simulink model "position_stabilization"  (R2018b)
settings: Solver=VariableStepAuto  StartTime=0.0  StopTime=10.0  RelTol=1e-3
values from neighbouring files (symbols this model uses):
  g = 9.8    [para.m]
  Ixx = 0.1    [para.m]
  m = 2    [para.m]
  x0 = zeros(6, 1)    [para.m]
settings Model: Creator=arthus  LastModifiedBy=longh

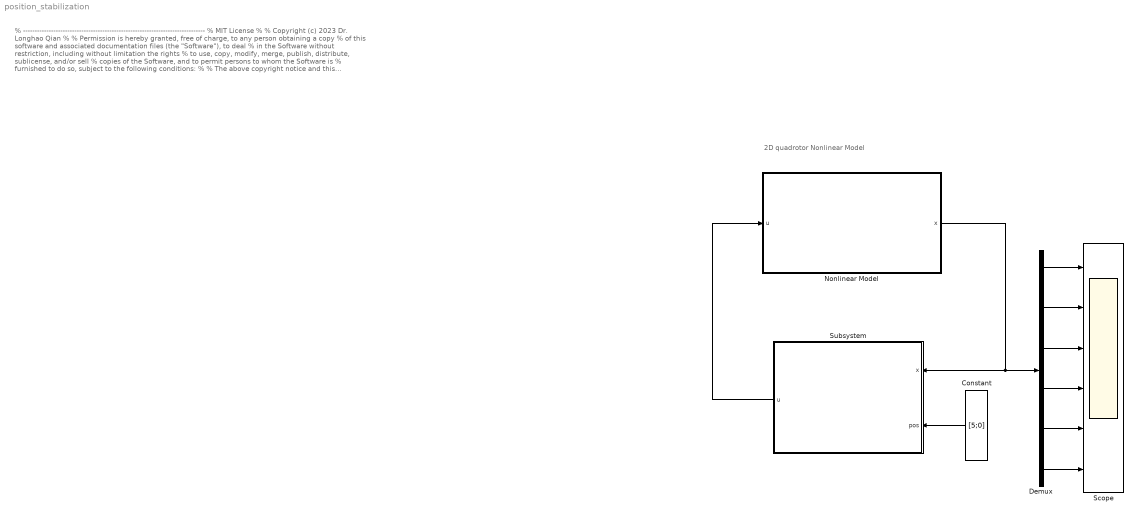
== system position_stabilization ==
  note: % ------------------------------------------------------------------------------
      | % MIT License
      | %
      | % Copyright (c) 2023 Dr. Longhao Qian
      | %
      | % Permission is hereby granted, free of charge, to any person obtaining a copy
      | % of this software and associated documentation files (the "Software"), to deal
      | % in the Software without restriction, including without limitation the rights
      | % to use, copy, modify, merge, publish, distribute, sublicense, and/or sell
      | % copies of the Software, and to permit persons to whom the Software is
      | % furnished to do so, subject to the following conditions:
      | %
      | % The above copyright notice and this permission notice shall be included in all
      | % copies or substantial portions of the Software.
      | %
      | % THE SOFTWARE IS PROVIDED "AS IS", WITHOUT WARRANTY OF ANY KIND, EXPRESS OR
      | % IMPLIED, INCLUDING BUT NOT LIMITED TO THE WARRANTIES OF MERCHANTABILITY,
      | % FITNESS FOR A PARTICULAR PURPOSE AND NONINFRINGEMENT. IN NO EVENT SHALL THE
      | % AUTHORS OR COPYRIGHT HOLDERS BE LIABLE FOR ANY CLAIM, DAMAGES OR OTHER
      | % LIABILITY, WHETHER IN AN ACTION OF CONTRACT, TORT OR OTHERWISE, ARISING FROM,
      | % OUT OF OR IN CONNECTION WITH THE SOFTWARE OR THE USE OR OTHER DEALINGS IN THE
      | % SOFTWARE.
      | % ------------------------------------------------------------------------------
  note: 2D quadrotor Nonlinear Model
  Constant : Constant  Value=[5;0]  VectorParams1D=off
  Demux : Demux  Outputs=6
  Nonlinear Model : Subsystem
  Scope : Scope  NumInputPorts=6
  Subsystem : Subsystem
  wires:
  Nonlinear Model/1(x) -> Subsystem/1(x), Demux/1
  Subsystem/1(u) -> Nonlinear Model/1(u)
  Demux/1 -> Scope/1
  Demux/2 -> Scope/2
  Demux/3 -> Scope/3
  Demux/4 -> Scope/4
  Demux/5 -> Scope/5
  Demux/6 -> Scope/6
  Constant/1 -> Subsystem/2(pos)

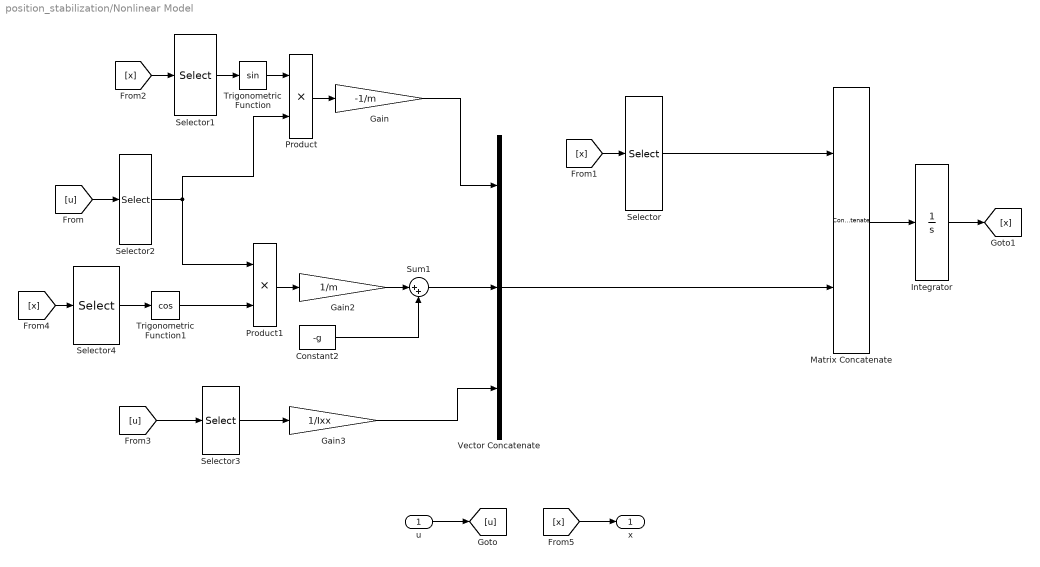
== system position_stabilization/Nonlinear Model ==
  u : Inport
  Constant2 : Constant  Value=-g
  Gain : Gain  Gain=-1/m
  Gain2 : Gain  Gain=1/m
  Gain3 : Gain  Gain=1/Ixx
  Integrator : Integrator  InitialCondition=x0
  Matrix Concatenate : Concatenate  Mode=Multidimensional array
  Product : Product
  Product1 : Product
  Selector : Selector  InputPortWidth=6  IndexOptions=Index vector (dialog)  Indices=[4 5 6]  OutputSizes=1
  Selector1 : Selector  InputPortWidth=6  IndexOptions=Index vector (dialog)  Indices=[3]  OutputSizes=1
  Selector2 : Selector  InputPortWidth=2  IndexOptions=Index vector (dialog)  Indices=[1]  OutputSizes=1
  Selector3 : Selector  InputPortWidth=2  IndexOptions=Index vector (dialog)  Indices=[2]  OutputSizes=1
  Selector4 : Selector  InputPortWidth=6  IndexOptions=Index vector (dialog)  Indices=[3]  OutputSizes=1
  Sum1 : Sum  Inputs=|++
  Trigonometric Function : Trigonometry
  Trigonometric Function1 : Trigonometry  Operator=cos
  Vector Concatenate : Concatenate  NumInputs=3  Mode=Multidimensional array
  x : Outport
  wires:
  Vector Concatenate/1 -> Matrix Concatenate/2
  Gain/1 -> Vector Concatenate/1
  Trigonometric Function/1 -> Product/1
  [x] -> x/1
  Integrator/1 -> [x]
  Product/1 -> Gain/1
  Selector2/1 -> Product1/1, Product/2
  [x] -> Selector4/1
  [u] -> Selector3/1
  [x] -> Selector/1
  Selector4/1 -> Trigonometric Function1/1
  Selector3/1 -> Gain3/1
  Sum1/1 -> Vector Concatenate/2
  Gain3/1 -> Vector Concatenate/3
  Product1/1 -> Gain2/1
  Selector1/1 -> Trigonometric Function/1
  Constant2/1 -> Sum1/2
  Trigonometric Function1/1 -> Product1/2
  [u] -> Selector2/1
  [x] -> Selector1/1
  Selector/1 -> Matrix Concatenate/1
  Matrix Concatenate/1 -> Integrator/1
  Gain2/1 -> Sum1/1
  u/1 -> [u]

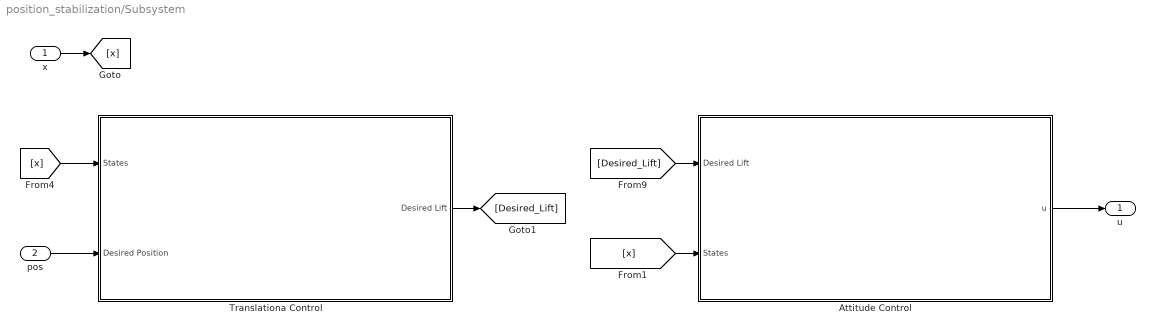
== system position_stabilization/Subsystem ==
  x : Inport
  pos : Inport  Port=2
  Attitude Control : Subsystem
  Translationa Control : Subsystem
  u : Outport
  wires:
  x/1 -> [x]
  [x] -> Attitude Control/2(States)
  pos/1 -> Translationa Control/2(Desired Position)
  [x] -> Translationa Control/1(States)
  Translationa Control/1(Desired Lift) -> [Desired_Lift]
  [Desired_Lift] -> Attitude Control/1(Desired Lift)
  Attitude Control/1(u) -> u/1

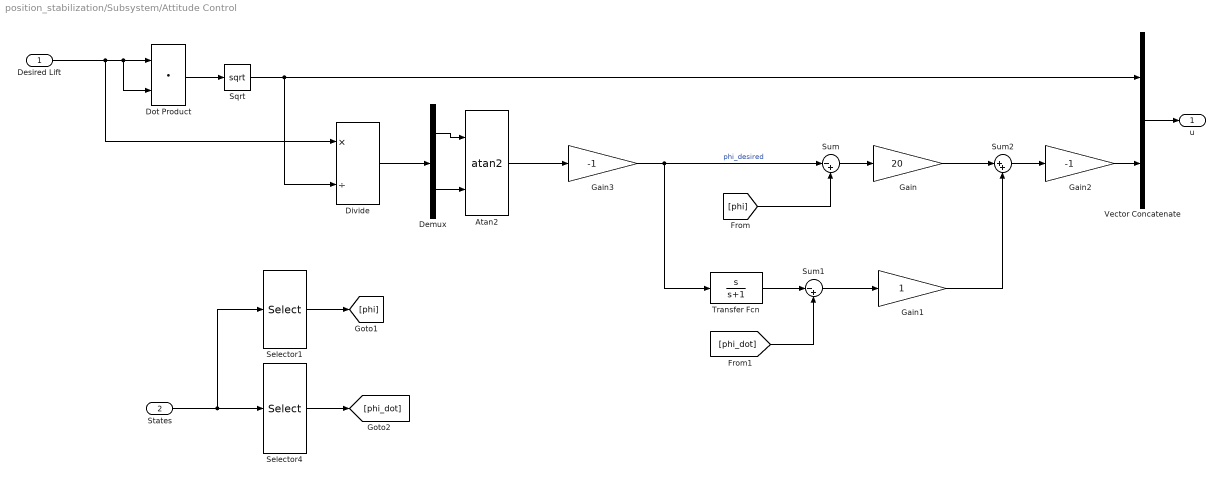
== system position_stabilization/Subsystem/Attitude Control ==
  Desired Lift : Inport
  States : Inport  Port=2
  Atan2 : Trigonometry  Operator=atan2
  Demux : Demux  Outputs=2
  Divide : Product  Inputs=*/
  Dot Product : DotProduct  InputSameDT=on  OutDataTypeStr=Inherit: Inherit via internal rule
  Gain : Gain  Gain=20
  Gain1 : Gain
  Gain2 : Gain  Gain=-1
  Gain3 : Gain  Gain=-1
  Selector1 : Selector  InputPortWidth=6  IndexOptions=Index vector (dialog)  Indices=[3]  OutputSizes=1
  Selector4 : Selector  InputPortWidth=6  IndexOptions=Index vector (dialog)  Indices=[6]  OutputSizes=1
  Sqrt : Sqrt  SaturateOnIntegerOverflow=on
  Sum : Sum  Inputs=|-+
  Sum1 : Sum  Inputs=|-+
  Sum2 : Sum  Inputs=|++
  Transfer Fcn : TransferFcn  Numerator=[1 0]  Denominator=[1 1]
  Vector Concatenate : Concatenate
  u : Outport
  wires:
  Selector1/1 -> [phi]
  States/1 -> Selector4/1, Selector1/1
  Selector4/1 -> [phi_dot]
  Desired Lift/1 -> Divide/1, Dot Product/2, Dot Product/1
  Dot Product/1 -> Sqrt/1
  Sqrt/1 -> Divide/2, Vector Concatenate/1
  Vector Concatenate/1 -> u/1
  Divide/1 -> Demux/1
  Atan2/1 -> Gain3/1
  [phi] -> Sum/2
  Sum/1 -> Gain/1
  Transfer Fcn/1 -> Sum1/1
  [phi_dot] -> Sum1/2
  Sum1/1 -> Gain1/1
  Gain/1 -> Sum2/1
  Gain1/1 -> Sum2/2
  Sum2/1 -> Gain2/1
  Gain2/1 -> Vector Concatenate/2
  Demux/1 -> Atan2/1
  Demux/2 -> Atan2/2
  Gain3/1 -> Transfer Fcn/1, Sum/1  "phi_desired"

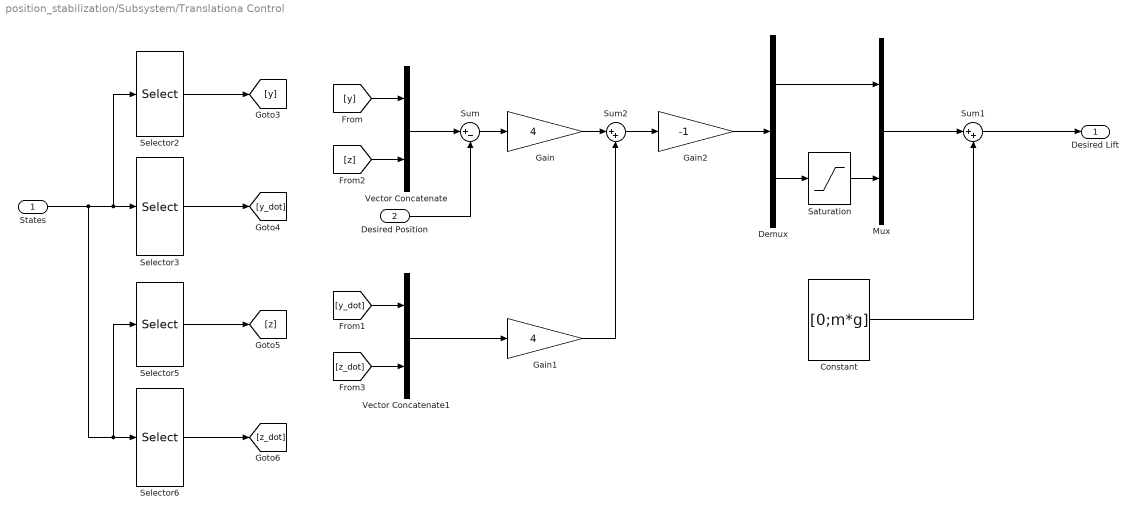
== system position_stabilization/Subsystem/Translationa Control ==
  States : Inport
  Desired Position : Inport  Port=2
  Constant : Constant  Value=[0;m*g]  VectorParams1D=off
  Demux : Demux  Outputs=2
  Gain : Gain  Gain=4
  Gain1 : Gain  Gain=4
  Gain2 : Gain  Gain=-1
  Mux : Mux  Inputs=2
  Saturation : Saturate  UpperLimit=inf  LowerLimit=-0.9 * m *g
  Selector2 : Selector  InputPortWidth=6  IndexOptions=Index vector (dialog)  Indices=[1]  OutputSizes=1
  Selector3 : Selector  InputPortWidth=6  IndexOptions=Index vector (dialog)  Indices=[4]  OutputSizes=1
  Selector5 : Selector  InputPortWidth=6  IndexOptions=Index vector (dialog)  Indices=[2]  OutputSizes=1
  Selector6 : Selector  InputPortWidth=6  IndexOptions=Index vector (dialog)  Indices=[5]  OutputSizes=1
  Sum : Sum  Inputs=|+-
  Sum1 : Sum  Inputs=|++
  Sum2 : Sum  Inputs=|++
  Vector Concatenate : Concatenate
  Vector Concatenate1 : Concatenate
  Desired Lift : Outport
  wires:
  Selector2/1 -> [y]
  Selector3/1 -> [y_dot]
  States/1 -> Selector6/1, Selector5/1, Selector3/1, Selector2/1
  Selector5/1 -> [z]
  Selector6/1 -> [z_dot]
  [z] -> Vector Concatenate/2
  [y] -> Vector Concatenate/1
  Vector Concatenate/1 -> Sum/1
  Desired Position/1 -> Sum/2
  Sum/1 -> Gain/1
  [y_dot] -> Vector Concatenate1/1
  [z_dot] -> Vector Concatenate1/2
  Constant/1 -> Sum1/2
  Sum1/1 -> Desired Lift/1
  Gain/1 -> Sum2/1
  Vector Concatenate1/1 -> Gain1/1
  Gain1/1 -> Sum2/2
  Sum2/1 -> Gain2/1
  Mux/1 -> Sum1/1
  Gain2/1 -> Demux/1
  Demux/1 -> Mux/1
  Demux/2 -> Saturation/1
  Saturation/1 -> Mux/2
